simulink model "SPIMaster_TMP123"  (R2016b)
settings: Solver=FixedStepDiscrete  StartTime=0.0  StopTime=10.0  FixedStep=1e-3  RelTol=1e-3
libraries: mbed_lib x5
settings Model: Creator=oh  LastModifiedBy=oh
settings OptimizationCC: DefaultParameterBehavior=Inlined
settings DebuggingCC: ParameterTunabilityLossMsg=error
settings HardwareCC: ProdBitPerPointer=32  ProdBitPerSizeT=32  ProdBitPerPtrDiffT=32  ProdLargestAtomicInteger=Long  ProdLargestAtomicFloat=Double  ProdWordSize=32  ProdHWDeviceType=ARM Compatible->ARM Cortex
settings RTWCC: SystemTargetFile=mbed.tlc  TemplateMakefile=mbed.tmf  Description=Mbed Target (Embedded Target)  GenerateReport=on  IncludeHyperlinkInReport=on  LaunchReport=on  TargetLang=C++  GenerateTraceInfo=on  GenerateTraceReport=on  GenerateTraceReportSl=on  GenerateTraceReportSf=on  GenerateTraceReportEml=on
settings CodeAppCC: ForceParamTrailComments=on  IgnoreCustomStorageClasses=off  OperatorAnnotations=on  SimulinkDataObjDesc=on  SFDataObjDesc=on  MATLABFcnDesc=on  InsertBlockDesc=on  MATLABSourceComments=on
settings STFCustomTargetCC: TargetLibSuffix=.a  TargetLangStandard=C++03 (ISO)  GenerateSampleERTMain=on  CombineOutputUpdateFcns=on  ERTCustomFileBanners=on  SupportContinuousTime=off  SupportNonInlinedSFcns=off  RemoveResetFunc=on  MATLABClassNameForMDSCustomization=Simulink.SoftwareTarget.ERTCustomization  GRTInterface=off  SystemTargetFile=mbed.tlc
settings ERTTargetCC: TargetLangStandard=C++03 (ISO)  GenerateSampleERTMain=on  ParMdlRefBuildCompliant=off  CompOptLevelCompliant=off  ConcurrentExecutionCompliant=off  ERTFirstTimeCompliant=off  ModelStepFunctionPrototypeControlCompliant=off  CPPClassGenCompliant=off  UseToolchainInfoCompliant=off  InlinedParameterPlacement=NonHierarchical  ERTCustomFileTemplate=mbed_file_process.tlc

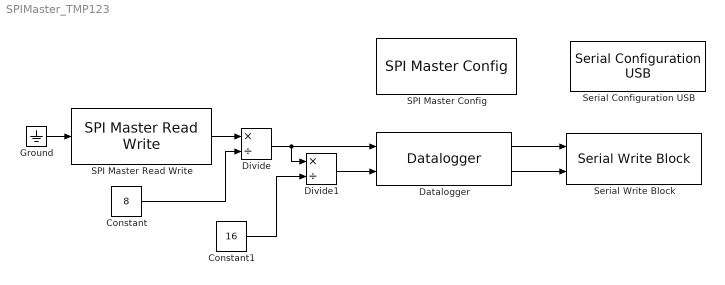
== system SPIMaster_TMP123 ==
  Constant : Constant  Value=8
  Constant1 : Constant  Value=16
  Datalogger : mbed_lib/Utilities/Datalogger  TypeInputPorts={ 'uint16' 1 'single' 1 }  TypeOfInputs={'1*uint16' '1*single'}  BufferSize=100  errEn=off  SampleTime=-1
  Divide : Product  Inputs=*/
  Divide1 : Product  Inputs=*/
  Ground : Ground
  SPI Master Config : mbed_lib/Serial/SPI/SPI Master Config  Priority=0  SPIPort=1  Freq=100000  Mode=0  Bits=8  MOSIPortNameShow=NC  MOSIPortName=0  MOSIPinNumber=7  MISOPortNameShow=A  MISOPortName=0  MISOPinNumber=6  SCLKPortName=A  Parameter13=0  SCLKPinNumber=5
  SPI Master Read Write : mbed_lib/Serial/SPI/SPI Master Read Write  SpiPort=1  CsPort=B  CsPin=6
  Serial Configuration USB : mbed_lib/Serial/UART/Serial Configuration USB  BaudRate=9600
  Serial Write Block : mbed_lib/Serial/UART/Serial Write Block  SerialPort=0  numData=on  SampleTime=-1
  wires:
  Ground/1 -> SPI Master Read Write/1
  SPI Master Read Write/1 -> Divide/1
  Constant/1 -> Divide/2
  Divide/1 -> Divide1/1, Datalogger/1
  Divide1/1 -> Datalogger/2
  Constant1/1 -> Divide1/2
  Datalogger/1 -> Serial Write Block/1
  Datalogger/2 -> Serial Write Block/2
